simulink model "SpaceRobotics_compare"  (R2024b)
settings: Solver=VariableStepAuto  StartTime=0.0  StopTime=10.0  RelTol=1e-3
values from neighbouring files (symbols this model uses):
  s = joint_angles_new - joint_angles    [inverse_kinematic_broyden.m]
  X = {r0x dr0x r0y dr0y theta0 dtheta0 theta1 dtheta1 theta2 dtheta2}    [Another_derivation_trail.m]
undefined symbols (not defined in the file or in its folder): Y, Z
libraries: sm_lib x23, nesl_utility x9
settings Model: Creator=Daniel  LastModifiedBy=admin

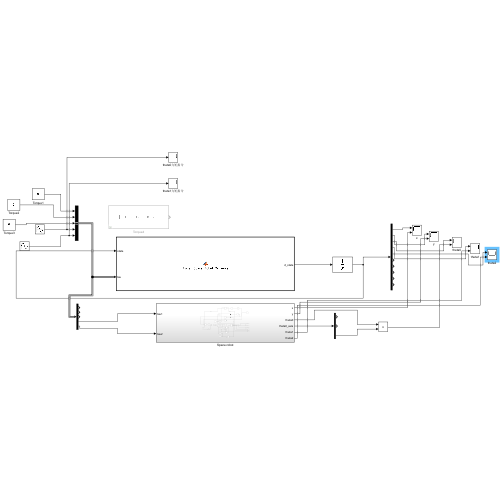
[thumbnail: Simulink's stored preview of the top-level diagram]
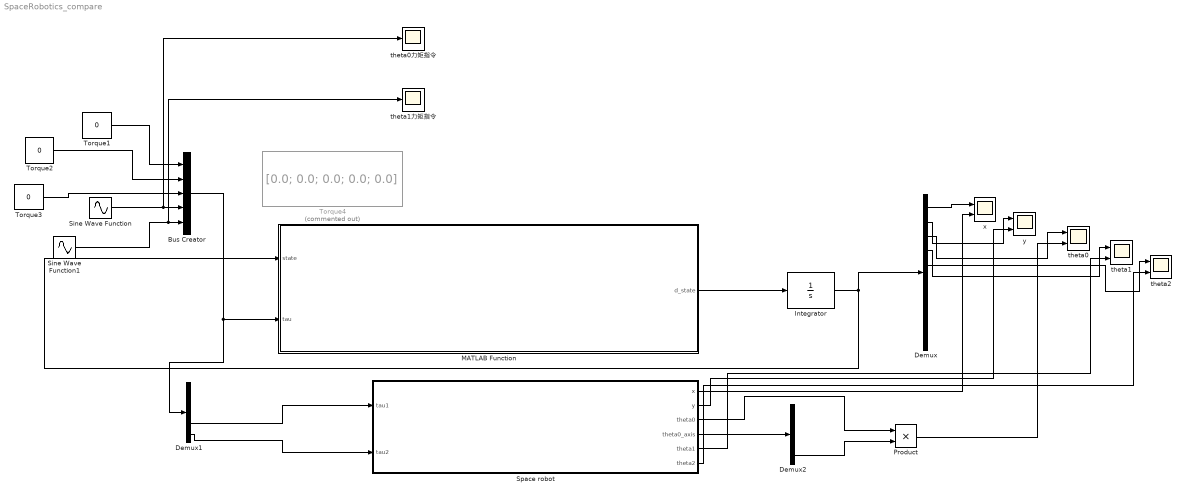
== system SpaceRobotics_compare ==
  Bus Creator : BusCreator  Inputs=5
  Demux : Demux  Outputs=10
  Demux1 : Demux  Outputs=5
  Demux2 : Demux  Outputs=3
  Integrator : Integrator  InitialCondition=[0.0; 0.0; 0.0; 0.0; 0.0; 0.0; 0.0; 0.0; 0.0; 0.0]
  MATLAB Function : MATLAB Function  TreatAsAtomicUnit=on
  Product : Product
  Sine Wave Function : Sin  SampleTime=0
  Sine Wave Function1 : Sin  Phase=pi/2  SampleTime=0
  Space robot : Subsystem
  Torque1 : Constant  Value=0
  Torque2 : Constant  Value=0
  Torque3 : Constant  Value=0
  Torque4 : Constant  Commented=on  Value=[0.0; 0.0; 0.0; 0.0; 0.0]
  theta0 : Scope  NumInputPorts=2
  theta0力矩指令 : Scope
  theta1 : Scope  NumInputPorts=2
  theta1力矩指令 : Scope
  theta2 : Scope  NumInputPorts=2
  x : Scope  NumInputPorts=2
  y : Scope  NumInputPorts=2
  wires:
  MATLAB Function/1(d_state) -> Integrator/1
  Integrator/1 -> MATLAB Function/1(state), Demux/1
  Bus Creator/1 -> Demux1/1, MATLAB Function/2(tau)
  Demux/1 -> x/1
  Demux/2 -> y/1
  Demux/3 -> theta0/1
  Demux/4 -> theta1/1
  Demux/5 -> theta2/1
  Demux1/5 -> Space robot/2(tau2)
  Demux1/4 -> Space robot/1(tau1)
  Space robot/1(x) -> x/2
  Space robot/2(y) -> y/2
  Space robot/5(theta1) -> theta1/2
  Space robot/6(theta2) -> theta2/2
  Torque1/1 -> Bus Creator/1
  Torque2/1 -> Bus Creator/2
  Torque3/1 -> Bus Creator/3
  Sine Wave Function/1 -> theta0力矩指令/1, Bus Creator/4
  Sine Wave Function1/1 -> theta1力矩指令/1, Bus Creator/5
  Space robot/4(theta0_axis) -> Demux2/1
  Demux2/3 -> Product/2
  Space robot/3(theta0) -> Product/1
  Product/1 -> theta0/2

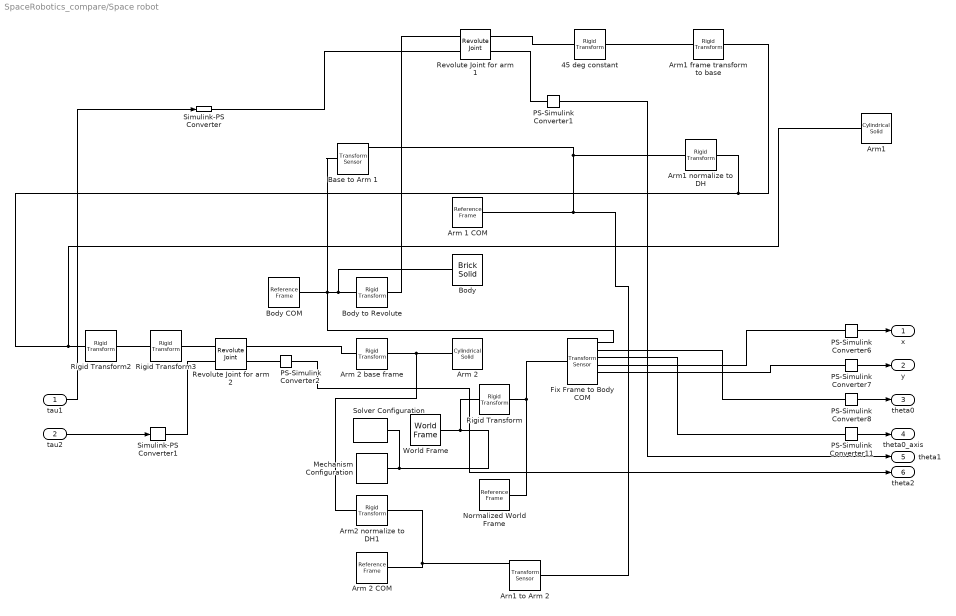
== system SpaceRobotics_compare/Space robot ==
  tau1 : Inport
  tau2 : Inport  Port=2
  45 deg constant : sm_lib/Frames and Transforms/Rigid Transform  RotationMethod=StandardAxis  FollAlignAxisA=+X  BaseAlignAxisA=+Y  FollAlignAxisB=+Y  BaseAlignAxisB=+Z  RotationStandardAxis=+Z  RotationAngle=45  RotationAngleUnits=deg  RotationArbitraryAxis=[0 0 1]  RotationSequenceAxes=FollowerAxes  RotationSequence=XYX  RotationSequenceAngles=[0 0 0]  RotationSequenceAnglesUnits=deg  RotationMatrix=[1 0 0;0 1 0;0 0 1]  Quaternion=[1 0 0 0]  TranslationMethod=Cartesian  TranslationCartesianOffset=[0 0 0]  TranslationCartesianOffsetUnits=m  TranslationStandardAxis=+Z  TranslationStandardOffset=0  TranslationStandardOffsetUnits=m  TranslationROffset=0  TranslationROffsetUnits=m  TranslationThetaOffset=0  TranslationThetaOffsetUnits=deg  TranslationZOffset=0  TranslationZOffsetUnits=m
  Arm 1 COM : sm_lib/Frames and Transforms/Reference Frame
  Arm 2 : sm_lib/Body Elements/Cylindrical Solid  CylinderRadius=0.12  CylinderRadiusUnits=m  CylinderLength=1  CylinderLengthUnits=m  ExportEntireGeometry=off  InertiaType=Custom  BasedOnType=Density  Density=1000  DensityUnits=kg/m^3  Mass=10  MassUnits=kg  CenterOfMass=[0 0 0]  CenterOfMassUnits=m  MomentsOfInertia=[2 2 2]  MomentsOfInertiaUnits=kg*m^2  ProductsOfInertia=[0 0 0]  ProductsOfInertiaUnits=kg*m^2  GraphicType=FromGeometry  MarkerShape=Sphere  MarkerSize=10  GraphicVisPropType=SimpleVisualProperties  GraphicDiffuseColor=[0.5 0.5 0.5]  GraphicOpacity=1  GraphicSpecularColor=[0.5 0.5 0.5 1.0]  GraphicAmbientColor=[0.15 0.15 0.15 1.0]  GraphicEmissiveColor=[0.0 0.0 0.0 1.0]  GraphicShininess=75  DoExposeReferenceFrame=on  SerializedFrames=<Frames/>
  Arm 2 COM : sm_lib/Frames and Transforms/Reference Frame
  Arm 2 base frame : sm_lib/Frames and Transforms/Rigid Transform  RotationMethod=StandardAxis  FollAlignAxisA=+X  BaseAlignAxisA=+Y  FollAlignAxisB=+Y  BaseAlignAxisB=+Z  RotationStandardAxis=+X  RotationAngle=90  RotationAngleUnits=deg  RotationArbitraryAxis=[0 0 1]  RotationSequenceAxes=FollowerAxes  RotationSequence=XYX  RotationSequenceAngles=[0 0 0]  RotationSequenceAnglesUnits=deg  RotationMatrix=[1 0 0;0 1 0;0 0 1]  Quaternion=[1 0 0 0]  TranslationMethod=Cartesian  TranslationCartesianOffset=[0 0 -0.5]  TranslationCartesianOffsetUnits=m  TranslationStandardAxis=+Z  TranslationStandardOffset=0  TranslationStandardOffsetUnits=m  TranslationROffset=0  TranslationROffsetUnits=m  TranslationThetaOffset=0  TranslationThetaOffsetUnits=deg  TranslationZOffset=0  TranslationZOffsetUnits=m
  Arm1 : sm_lib/Body Elements/Cylindrical Solid  CylinderRadius=0.12  CylinderRadiusUnits=m  CylinderLength=1  CylinderLengthUnits=m  ExportEntireGeometry=off  InertiaType=Custom  BasedOnType=Density  Density=1000  DensityUnits=kg/m^3  Mass=10  MassUnits=kg  CenterOfMass=[0 0 0]  CenterOfMassUnits=m  MomentsOfInertia=[2 2 2]  MomentsOfInertiaUnits=kg*m^2  ProductsOfInertia=[0 0 0]  ProductsOfInertiaUnits=kg*m^2  GraphicType=FromGeometry  MarkerShape=Sphere  MarkerSize=10  GraphicVisPropType=SimpleVisualProperties  GraphicDiffuseColor=[0.5 0.5 0.5]  GraphicOpacity=1  GraphicSpecularColor=[0.5 0.5 0.5 1.0]  GraphicAmbientColor=[0.15 0.15 0.15 1.0]  GraphicEmissiveColor=[0.0 0.0 0.0 1.0]  GraphicShininess=75  DoExposeReferenceFrame=on  SerializedFrames=<Frames/>
  Arm1 frame transform to base : sm_lib/Frames and Transforms/Rigid Transform  RotationMethod=StandardAxis  FollAlignAxisA=+X  BaseAlignAxisA=+Y  FollAlignAxisB=+Y  BaseAlignAxisB=+Z  RotationStandardAxis=+X  RotationAngle=90  RotationAngleUnits=deg  RotationArbitraryAxis=[0 0 1]  RotationSequenceAxes=FollowerAxes  RotationSequence=XYX  RotationSequenceAngles=[0 0 0]  RotationSequenceAnglesUnits=deg  RotationMatrix=[1 0 0;0 1 0;0 0 1]  Quaternion=[1 0 0 0]  TranslationMethod=Cartesian  TranslationCartesianOffset=[0 0 -0.5]  TranslationCartesianOffsetUnits=m  TranslationStandardAxis=+Z  TranslationStandardOffset=0  TranslationStandardOffsetUnits=m  TranslationROffset=0  TranslationROffsetUnits=m  TranslationThetaOffset=0  TranslationThetaOffsetUnits=deg  TranslationZOffset=0  TranslationZOffsetUnits=m
  Arm1 normalize to DH : sm_lib/Frames and Transforms/Rigid Transform  RotationMethod=RotationMatrix  FollAlignAxisA=+X  BaseAlignAxisA=+Y  FollAlignAxisB=+Y  BaseAlignAxisB=+Z  RotationStandardAxis=+X  RotationAngle=90  RotationAngleUnits=deg  RotationArbitraryAxis=[0 0 1]  RotationSequenceAxes=FollowerAxes  RotationSequence=XYX  RotationSequenceAngles=[0 0 0]  RotationSequenceAnglesUnits=deg  RotationMatrix=[0 0 1;-1 0 0;0 -1 0]  Quaternion=[1 0 0 0]  TranslationMethod=None  TranslationCartesianOffset=[0 0 0]  TranslationCartesianOffsetUnits=m  TranslationStandardAxis=+Z  TranslationStandardOffset=0  TranslationStandardOffsetUnits=m  TranslationROffset=0  TranslationROffsetUnits=m  TranslationThetaOffset=0  TranslationThetaOffsetUnits=deg  TranslationZOffset=0  TranslationZOffsetUnits=m
  Arm2 normalize to DH1 : sm_lib/Frames and Transforms/Rigid Transform  RotationMethod=RotationMatrix  FollAlignAxisA=+X  BaseAlignAxisA=+Y  FollAlignAxisB=+Y  BaseAlignAxisB=+Z  RotationStandardAxis=+X  RotationAngle=90  RotationAngleUnits=deg  RotationArbitraryAxis=[0 0 1]  RotationSequenceAxes=FollowerAxes  RotationSequence=XYX  RotationSequenceAngles=[0 0 0]  RotationSequenceAnglesUnits=deg  RotationMatrix=[0 0 1;-1 0 0;0 -1 0]  Quaternion=[1 0 0 0]  TranslationMethod=None  TranslationCartesianOffset=[0 0 0]  TranslationCartesianOffsetUnits=m  TranslationStandardAxis=+Z  TranslationStandardOffset=0  TranslationStandardOffsetUnits=m  TranslationROffset=0  TranslationROffsetUnits=m  TranslationThetaOffset=0  TranslationThetaOffsetUnits=deg  TranslationZOffset=0  TranslationZOffsetUnits=m
  Arn1 to Arm 2 : sm_lib/Frames and Transforms/Transform Sensor  MeasurementFrame=Base  RotationSequence=XYX  SenseAngle=on  SenseAxis=on  SenseQ=off  SenseR=off  SenseRotationSequence=off  SenseOmegaX=off  SenseOmegaY=off  SenseOmegaZ=off  SenseOmega=off  SenseQDot=off  SenseRDot=off  SenseRotationSequenceDot=off  SenseAlphaX=off  SenseAlphaY=off  SenseAlphaZ=off  SenseAlpha=off  SenseQDDot=off  SenseRDDot=off  SenseX=off  SenseY=off  SenseZ=off  SenseXYZ=off  SenseRad=off  SenseAzim=off  SenseDist=off  SenseInc=off  SenseXDot=off  SenseYDot=off  SenseZDot=off  SenseXYZDot=off  SenseRadDot=off  SenseAzimDot=off  SenseDistDot=off  SenseIncDot=off  SenseXDDot=off  SenseYDDot=off  SenseZDDot=off  SenseXYZDDot=off  SenseRadDDot=off  SenseAzimDDot=off  SenseDistDDot=off  SenseIncDDot=off
  Base to Arm 1 : sm_lib/Frames and Transforms/Transform Sensor  MeasurementFrame=Base  RotationSequence=XYX  SenseAngle=on  SenseAxis=on  SenseQ=off  SenseR=off  SenseRotationSequence=off  SenseOmegaX=off  SenseOmegaY=off  SenseOmegaZ=off  SenseOmega=off  SenseQDot=off  SenseRDot=off  SenseRotationSequenceDot=off  SenseAlphaX=off  SenseAlphaY=off  SenseAlphaZ=off  SenseAlpha=off  SenseQDDot=off  SenseRDDot=off  SenseX=off  SenseY=off  SenseZ=off  SenseXYZ=off  SenseRad=off  SenseAzim=off  SenseDist=off  SenseInc=off  SenseXDot=off  SenseYDot=off  SenseZDot=off  SenseXYZDot=off  SenseRadDot=off  SenseAzimDot=off  SenseDistDot=off  SenseIncDot=off  SenseXDDot=off  SenseYDDot=off  SenseZDDot=off  SenseXYZDDot=off  SenseRadDDot=off  SenseAzimDDot=off  SenseDistDDot=off  SenseIncDDot=off
  Body : sm_lib/Body Elements/Brick Solid  BrickDimensions=[1 1 1]  BrickDimensionsUnits=m  ExportEntireGeometry=off  InertiaType=CalculateFromGeometry  BasedOnType=Density  Density=500  DensityUnits=kg/m^3  Mass=1  MassUnits=kg  CenterOfMass=[0 0 0]  CenterOfMassUnits=m  MomentsOfInertia=[1 1 1]  MomentsOfInertiaUnits=kg*m^2  ProductsOfInertia=[0 0 0]  ProductsOfInertiaUnits=kg*m^2  GraphicType=FromGeometry  MarkerShape=Sphere  MarkerSize=10  GraphicVisPropType=SimpleVisualProperties  GraphicDiffuseColor=[0.5 0.5 0.5]  GraphicOpacity=1  GraphicSpecularColor=[0.5 0.5 0.5 1.0]  GraphicAmbientColor=[0.15 0.15 0.15 1.0]  GraphicEmissiveColor=[0.0 0.0 0.0 1.0]  GraphicShininess=75  DoExposeReferenceFrame=on  SerializedFrames=<Frames><Frame><Id>Frame1</Id><Value><Name>F1</Name><Origin><Source>CenterOfMassFrame</Source><FeatureName></FeatureName></Origin><PrimaryAxis><DefinedDirection>+Z</DefinedDirection><Source>ReferenceFrame</Source><SourceDirection>+Z</SourceDirection><FeatureName></FeatureName></PrimaryAxis><SecondaryAxis><DefinedDirection>+X</DefinedDirection><Source>ReferenceFrame</Source><SourceDirection>+X</SourceDirection><FeatureName></FeatureName></SecondaryAxis></Value></Frame></Frames>
  Body COM : sm_lib/Frames and Transforms/Reference Frame
  Body to Revolute : sm_lib/Frames and Transforms/Rigid Transform  RotationMethod=None  FollAlignAxisA=+X  BaseAlignAxisA=+Y  FollAlignAxisB=+Y  BaseAlignAxisB=+Z  RotationStandardAxis=+X  RotationAngle=90  RotationAngleUnits=deg  RotationArbitraryAxis=[0 0 1]  RotationSequenceAxes=FollowerAxes  RotationSequence=XYX  RotationSequenceAngles=[0 0 0]  RotationSequenceAnglesUnits=deg  RotationMatrix=[1 0 0;0 1 0;0 0 1]  Quaternion=[1 0 0 0]  TranslationMethod=Cartesian  TranslationCartesianOffset=[0.5 0.5 0]  TranslationCartesianOffsetUnits=m  TranslationStandardAxis=+Z  TranslationStandardOffset=0  TranslationStandardOffsetUnits=m  TranslationROffset=0  TranslationROffsetUnits=m  TranslationThetaOffset=0  TranslationThetaOffsetUnits=deg  TranslationZOffset=0  TranslationZOffsetUnits=m
  Fix Frame to Body COM : sm_lib/Frames and Transforms/Transform Sensor  MeasurementFrame=World  RotationSequence=XYX  SenseAngle=on  SenseAxis=on  SenseQ=off  SenseR=off  SenseRotationSequence=off  SenseOmegaX=off  SenseOmegaY=off  SenseOmegaZ=off  SenseOmega=off  SenseQDot=off  SenseRDot=off  SenseRotationSequenceDot=off  SenseAlphaX=off  SenseAlphaY=off  SenseAlphaZ=off  SenseAlpha=off  SenseQDDot=off  SenseRDDot=off  SenseX=on  SenseY=on  SenseZ=off  SenseXYZ=on  SenseRad=off  SenseAzim=off  SenseDist=off  SenseInc=off  SenseXDot=off  SenseYDot=off  SenseZDot=off  SenseXYZDot=off  SenseRadDot=off  SenseAzimDot=off  SenseDistDot=off  SenseIncDot=off  SenseXDDot=off  SenseYDDot=off  SenseZDDot=off  SenseXYZDDot=off  SenseRadDDot=off  SenseAzimDDot=off  SenseDistDDot=off  SenseIncDDot=off
  Mechanism Configuration : sm_lib/Utilities/Mechanism Configuration  UniformGravity=Constant  GravityVector=[0 0 0]  GravityVectorUnits=m/s^2  LinearizationDelta=0.001  JointModeTransitionNonlinearIterations=100
  Normalized World Frame : sm_lib/Frames and Transforms/Reference Frame
  PS-Simulink Converter{1..2,6..8,11} (6 alike) : nesl_utility/PS-Simulink Converter  PhysicalDomain=network_engine_domain  SubClassName=ps_output  LeftPortType=input  RightPortType=output  PseudoPeriodic=off  Frequencies=[]  VectorFormat=inherit  Unit=inherit  AffineConversion=off
  Revolute Joint for arm 1 : sm_lib/Joints/Revolute Joint  JointMode=Normal  CompositeWrenchDir=BaseOnFollower  CompositeWrenchFrame=BaseFrame  SenseConstraintForce=off  SenseConstraintTorque=off  SenseTotalForce=off  SenseTotalTorque=off  PositionTargetSpecify=on  PositionTargetPriority=High  PositionTargetValue=0  PositionTargetValueUnits=deg  VelocityTargetSpecify=off  VelocityTargetPriority=High  VelocityTargetValue=0  VelocityTargetValueUnits=deg/s  EquilibriumPosition=0  EquilibriumPositionUnits=deg  SpringStiffness=0  SpringStiffnessUnits=N*m/deg  DampingCoefficient=0  DampingCoefficientUnits=N*m/(deg/s)  LowerLimitSpecify=off  LowerLimitBound=-90  LowerLimitBoundUnits=deg  LowerLimitStiffness=1e4  LowerLimitStiffnessUnits=N*m/deg  LowerLimitDamping=10  LowerLimitDampingUnits=N*m/(deg/s)  LowerLimitTransitionRegionWidth=0.1  LowerLimitTransitionRegionWidthUnits=deg  UpperLimitSpecify=off  UpperLimitBound=90  UpperLimitBoundUnits=deg  UpperLimitStiffness=1e4  UpperLimitStiffnessUnits=N*m/deg  UpperLimitDamping=10  UpperLimitDampingUnits=N*m/(deg/s)  UpperLimitTransitionRegionWidth=0.1  UpperLimitTransitionRegionWidthUnits=deg  TorqueActuationMode=InputTorque  MotionActuationMode=ComputedMotion  SensePosition=on  SenseVelocity=off  SenseAcceleration=off  SenseTorqueForce=off  SenseLowerLimitTorqueForce=off  SenseUpperLimitTorqueForce=off
  Revolute Joint for arm 2 : sm_lib/Joints/Revolute Joint  JointMode=Normal  CompositeWrenchDir=BaseOnFollower  CompositeWrenchFrame=BaseFrame  SenseConstraintForce=off  SenseConstraintTorque=off  SenseTotalForce=off  SenseTotalTorque=off  PositionTargetSpecify=on  PositionTargetPriority=High  PositionTargetValue=0  PositionTargetValueUnits=deg  VelocityTargetSpecify=off  VelocityTargetPriority=High  VelocityTargetValue=0  VelocityTargetValueUnits=deg/s  EquilibriumPosition=0  EquilibriumPositionUnits=deg  SpringStiffness=0  SpringStiffnessUnits=N*m/deg  DampingCoefficient=0  DampingCoefficientUnits=N*m/(deg/s)  LowerLimitSpecify=off  LowerLimitBound=-90  LowerLimitBoundUnits=deg  LowerLimitStiffness=1e4  LowerLimitStiffnessUnits=N*m/deg  LowerLimitDamping=10  LowerLimitDampingUnits=N*m/(deg/s)  LowerLimitTransitionRegionWidth=0.1  LowerLimitTransitionRegionWidthUnits=deg  UpperLimitSpecify=off  UpperLimitBound=90  UpperLimitBoundUnits=deg  UpperLimitStiffness=1e4  UpperLimitStiffnessUnits=N*m/deg  UpperLimitDamping=10  UpperLimitDampingUnits=N*m/(deg/s)  UpperLimitTransitionRegionWidth=0.1  UpperLimitTransitionRegionWidthUnits=deg  TorqueActuationMode=InputTorque  MotionActuationMode=ComputedMotion  SensePosition=on  SenseVelocity=off  SenseAcceleration=off  SenseTorqueForce=off  SenseLowerLimitTorqueForce=off  SenseUpperLimitTorqueForce=off
  Rigid Transform : sm_lib/Frames and Transforms/Rigid Transform  RotationMethod=StandardAxis  FollAlignAxisA=+X  BaseAlignAxisA=+Y  FollAlignAxisB=+Y  BaseAlignAxisB=+Z  RotationStandardAxis=+Z  RotationAngle=-45  RotationAngleUnits=deg  RotationArbitraryAxis=[0 0 1]  RotationSequenceAxes=FollowerAxes  RotationSequence=XYX  RotationSequenceAngles=[0 0 0]  RotationSequenceAnglesUnits=deg  RotationMatrix=[1 0 0;0 1 0;0 0 1]  Quaternion=[1 0 0 0]  TranslationMethod=Cartesian  TranslationCartesianOffset=[-1.20711 0 0]  TranslationCartesianOffsetUnits=m  TranslationStandardAxis=+Z  TranslationStandardOffset=0  TranslationStandardOffsetUnits=m  TranslationROffset=0  TranslationROffsetUnits=m  TranslationThetaOffset=0  TranslationThetaOffsetUnits=deg  TranslationZOffset=0  TranslationZOffsetUnits=m
  Rigid Transform2 : sm_lib/Frames and Transforms/Rigid Transform  RotationMethod=StandardAxis  FollAlignAxisA=+X  BaseAlignAxisA=+Y  FollAlignAxisB=+Y  BaseAlignAxisB=+Z  RotationStandardAxis=+Z  RotationAngle=0  RotationAngleUnits=deg  RotationArbitraryAxis=[0 0 1]  RotationSequenceAxes=FollowerAxes  RotationSequence=XYX  RotationSequenceAngles=[0 0 0]  RotationSequenceAnglesUnits=deg  RotationMatrix=[1 0 0;0 1 0;0 0 1]  Quaternion=[1 0 0 0]  TranslationMethod=Cartesian  TranslationCartesianOffset=[0 0 0.5]  TranslationCartesianOffsetUnits=m  TranslationStandardAxis=+Z  TranslationStandardOffset=0  TranslationStandardOffsetUnits=m  TranslationROffset=0  TranslationROffsetUnits=m  TranslationThetaOffset=0  TranslationThetaOffsetUnits=deg  TranslationZOffset=0  TranslationZOffsetUnits=m
  Rigid Transform3 : sm_lib/Frames and Transforms/Rigid Transform  RotationMethod=StandardAxis  FollAlignAxisA=+X  BaseAlignAxisA=+Y  FollAlignAxisB=+Y  BaseAlignAxisB=+Z  RotationStandardAxis=+X  RotationAngle=90  RotationAngleUnits=deg  RotationArbitraryAxis=[0 0 1]  RotationSequenceAxes=FollowerAxes  RotationSequence=XYX  RotationSequenceAngles=[0 0 0]  RotationSequenceAnglesUnits=deg  RotationMatrix=[1 0 0;0 1 0;0 0 1]  Quaternion=[1 0 0 0]  TranslationMethod=Cartesian  TranslationCartesianOffset=[0 0 0]  TranslationCartesianOffsetUnits=m  TranslationStandardAxis=+Z  TranslationStandardOffset=0  TranslationStandardOffsetUnits=m  TranslationROffset=0  TranslationROffsetUnits=m  TranslationThetaOffset=0  TranslationThetaOffsetUnits=deg  TranslationZOffset=0  TranslationZOffsetUnits=m
  Simulink-PS Converter : nesl_utility/Simulink-PS Converter  PhysicalDomain=network_engine_domain  SubClassName=ps_input  LeftPortType=input  RightPortType=output  PseudoPeriodic=off  Frequencies=[]  NoiseDistribution=none  NoiseParameters=[]  Unit=1  AffineConversion=off  FilteringAndDerivatives=provide  SimscapeFilterOrder=1  InputFilterTimeConstant=0.001  UdotUserProvided=0
  Simulink-PS Converter1 : nesl_utility/Simulink-PS Converter  PhysicalDomain=network_engine_domain  SubClassName=ps_input  LeftPortType=input  RightPortType=output  PseudoPeriodic=off  Frequencies=[]  NoiseDistribution=none  NoiseParameters=[]  Unit=1  AffineConversion=off  FilteringAndDerivatives=provide  SimscapeFilterOrder=1  InputFilterTimeConstant=0.001  UdotUserProvided=0
  Solver Configuration : nesl_utility/Solver Configuration  PhysicalDomain=network_engine_domain  SubClassName=solver  LeftPortType=input  RightPortType=generic  Tones=[]  Harmonics=[]  SimulateNoise=off  Profile=off  UseLocalSampling=off  EnableSwitchedLinearOptims=on  FrequencyDomain=off  UseCCode=off  RelTol=0.001  AbsTol=0.001  MinStep=1e-09  ToWorkspace=off  RevertToSquareIcSolve=off  NumHomotopyIterations=100  PhasorMode=off  PhasorModeNumHarmonics=1  ConsistencySolver=NEWTON_XTOL_AFTER_FTOL  IndexReductionMethod=DerivativeReplacement  DoDC=off  ResidualTolerance=1e-09  ConsistencyTolSource=GLOBAL  ConsistencyAbsTol=0.001  ConsistencyRelTol=0.001  ConsistencyTolFactor=0.001  UseLocalSolver=off  LocalSolverChoice=NE_BACKWARD_EULER_ADVANCER  ResolveIndetEquations=on  FunctionEvalNumThread=1  LocalSolverSampleTime=0.001  DoFixedCost=off  MaxNonlinIter=3  MaxModeIter=2  ComputeImpulses=off  ImpulseIterations=2  LinearAlgebra=auto  LinearAlgebraNumThread=0  EquationFormulation=NE_TIME_EF  DelaysMemoryBudget=1024  AutomaticFiltering=on  FilteringTimeConstant=0.001  PartitionStorageMethod=AS_NEEDED  PartitionMemoryBudget=1024  PartitionMethod=ROBUST  MultibodyUseLocalSolver=off  MultibodyLocalSolverChoice=ODE1  MultibodyLocalSolverSampleTime=0.001
  World Frame : sm_lib/Frames and Transforms/World Frame
  x : Outport
  y : Outport  Port=2
  theta0 : Outport  Port=3
  theta0_axis : Outport  Port=4
  theta1 : Outport  Port=5
  theta2 : Outport  Port=6
  wires:
  PS-Simulink Converter1/1 -> theta1/1
  tau2/1 -> Simulink-PS Converter1/1
  tau1/1 -> Simulink-PS Converter/1
  PS-Simulink Converter7/1 -> y/1
  PS-Simulink Converter8/1 -> theta0/1
  PS-Simulink Converter11/1 -> theta0_axis/1
  PS-Simulink Converter6/1 -> x/1
  PS-Simulink Converter2/1 -> theta2/1
  connections:
  Rigid Transform3/RConn1 -- Revolute Joint for arm 2/LConn1
  Arn1 to Arm 2/LConn1 -- Arm 1 COM/RConn1 -- Arm1 normalize to DH/LConn1 -- Base to Arm 1/RConn1
  Revolute Joint for arm 2/RConn1 -- Arm 2 base frame/RConn1
  Arm1/RConn1 -- Arm1 frame transform to base/LConn1 -- Arm1 normalize to DH/RConn1 -- Rigid Transform2/LConn1
  Rigid Transform2/RConn1 -- Rigid Transform3/LConn1
  PS-Simulink Converter6/LConn1 -- Fix Frame to Body COM/RConn4
  PS-Simulink Converter7/LConn1 -- Fix Frame to Body COM/RConn5
  Simulink-PS Converter/RConn1 -- Revolute Joint for arm 1/LConn2
  Simulink-PS Converter1/RConn1 -- Revolute Joint for arm 2/LConn2
  Body to Revolute/LConn1 -- Base to Arm 1/LConn1 -- Body COM/RConn1 -- Fix Frame to Body COM/RConn1 -- Body/RConn1
  Arm2 normalize to DH1/LConn1 -- Arm 2 COM/RConn1 -- Arn1 to Arm 2/RConn1
  Revolute Joint for arm 1/RConn2 -- PS-Simulink Converter1/LConn1
  World Frame/RConn1 -- Solver Configuration/RConn1 -- Mechanism Configuration/RConn1 -- Rigid Transform/LConn1
  Rigid Transform/RConn1 -- Fix Frame to Body COM/LConn1 -- Normalized World Frame/RConn1
  PS-Simulink Converter8/LConn1 -- Fix Frame to Body COM/RConn2
  Body to Revolute/RConn1 -- Revolute Joint for arm 1/LConn1
  Arm 2 base frame/LConn1 -- Arm2 normalize to DH1/RConn1 -- Arm 2/RConn1
  Revolute Joint for arm 1/RConn1 -- 45 deg constant/RConn1
  45 deg constant/LConn1 -- Arm1 frame transform to base/RConn1
  Fix Frame to Body COM/RConn3 -- PS-Simulink Converter11/LConn1
  PS-Simulink Converter2/LConn1 -- Revolute Joint for arm 2/RConn2

== matlab function SpaceRobotics_compare/MATLAB Function ==
  data: d_state output; state input; tau input
function d_state = Planar_Space_Robot_Dynamics(state, tau)
    % Explicit definition of dynamic constants
    robot_dynamics_constants.m0 = 500;
    robot_dynamics_constants.m1 = 10;
    robot_dynamics_constants.m2 = 10;
    robot_dynamics_constants.b0 = sqrt(0.5^2 + 0.5^2);
    robot_dynamics_constants.l1 = 1;
    robot_dynamics_constants.l2 = 1;
    robot_dynamics_constants.Ic0 = 83.3333;
    robot_dynamics_constants.Ic1 = 2;
    robot_dynamics_constants.Ic2 = 2;

    normalized_theta0 = mod(state(3), 2*pi);
    normalized_theta1 = mod(state(4), 2*pi);
    normalized_theta2 = mod(state(5), 2*pi);
    q = state(1:5);
    q(3) = normalized_theta0;
    q(4) = normalized_theta1;
    q(5) = normalized_theta2;
    q_dot = state(6:10);
    
    [inertial_term_matrix, coriolis_term] = Get_Planar_Dynamic_Matrix(q, q_dot, robot_dynamics_constants);
    %Dq = tau - coriolis_term;
    Dq = tau - coriolis_term;

    q_ddot = inertial_term_matrix \ Dq;

    d_state = [q_dot; q_ddot];
end

% Man fuck finally it matches hahahahahahahaha

function [H, F] = Get_Planar_Dynamic_Matrix(state_vector, state_dot, robot_dynamics_constants)
    % state_vector = [r0x, r0y, theta0, theta1, theta2]
    % state_dot = [r0x_dot, r0y_dot, theta0_dot, theta1_dot, theta2_dot]
    % Planar space robot dynamics
    % angles
    theta0 = state_vector(3);
    theta1 = state_vector(4);
    theta2 = state_vector(5);
    theta0_dot = state_dot(3);
    theta1_dot = state_dot(4);
    theta2_dot = state_dot(5);
    c0 = cos(theta0);
    c1 = cos(theta1);
    c2 = cos(theta2);
    c01 = cos(theta0 + theta1);
    c02 = cos(theta0 + theta2);
    c12 = cos(theta1 + theta2);
    c012 = cos(theta0 + theta1 + theta2);
    s0 = sin(theta0);
    s1 = sin(theta1);
    s2 = sin(theta2);
    s01 = sin(theta0 + theta1);
    s02 = sin(theta0 + theta2);
    s12 = sin(theta1 + theta2);
    s012 = sin(theta0 + theta1 + theta2);

    m_0 = robot_dynamics_constants.m0;
    m_1 = robot_dynamics_constants.m1;
    m_2 = robot_dynamics_constants.m2;
    b_0 = robot_dynamics_constants.b0;
    l_1 = robot_dynamics_constants.l1;
    l_2 = robot_dynamics_constants.l2;
    I_c0 = robot_dynamics_constants.Ic0;
    I_c1 = robot_dynamics_constants.Ic1;
    I_c2 = robot_dynamics_constants.Ic2;



    % Define the h matrix elements based on the equations provided
    h11 = m_0 + m_1 + m_2;
    h12 = 0;
    h13 = - (m_1*(2*b_0*s0 + l_1*s01))/2 - (m_2*(2*b_0*s0 + 2*l_1*s01 + l_2*s012))/2;
    h14 = - (m_2*(2*l_1*s01 + l_2*s012))/2 - (l_1*m_1*s01)/2;
    h15 = -(l_2*m_2*s012)/2;
    
    h21 = 0;
    h22 = m_0 + m_1 + m_2;
    h23 = (m_1*(2*b_0*c0 + c01*l_1))/2 + (m_2*(2*b_0*c0 + 2*c01*l_1 + c012*l_2))/2;
    h24 = (m_2*(2*c01*l_1 + c012*l_2))/2 + (c01*l_1*m_1)/2;
    h25 = (c012*l_2*m_2)/2;
    
    h31 = - m_1*(b_0*s0 + (l_1*s01)/2) - m_2*(b_0*s0 + l_1*s01 + (l_2*s012)/2);
    h32 = m_1*(b_0*c0 + (c01*l_1)/2) + m_2*(b_0*c0 + c01*l_1 + (c012*l_2)/2);
    h33 = I_c0 + I_c1 + I_c2 + m_2*(b_0*c0 + c01*l_1 + (c012*l_2)/2)^2 + m_2*(b_0*s0 + l_1*s01 + (l_2*s012)/2)^2 + m_1*(b_0*c0 + (c01*l_1)/2)^2 + m_1*(b_0*s0 + (l_1*s01)/2)^2;
    h34 = I_c1 + I_c2 + m_2*(c01*l_1 + (c012*l_2)/2)*(b_0*c0 + c01*l_1 + (c012*l_2)/2) + m_2*(l_1*s01 + (l_2*s012)/2)*(b_0*s0 + l_1*s01 + (l_2*s012)/2) + (c01*l_1*m_1*(b_0*c0 + (c01*l_1)/2))/2 + (l_1*m_1*s01*(b_0*s0 + (l_1*s01)/2))/2;
    h35 = I_c2 + (c012*l_2*m_2*(b_0*c0 + c01*l_1 + (c012*l_2)/2))/2 + (l_2*m_2*s012*(b_0*s0 + l_1*s01 + (l_2*s012)/2))/2;
    
    h41 = - m_2*(l_1*s01 + (l_2*s012)/2) - (l_1*m_1*s01)/2;
    h42 = m_2*(c01*l_1 + (c012*l_2)/2) + (c01*l_1*m_1)/2;
    h43 = I_c1 + I_c2 + m_2*(c01*l_1 + (c012*l_2)/2)*(b_0*c0 + c01*l_1 + (c012*l_2)/2) + m_2*(l_1*s01 + (l_2*s012)/2)*(b_0*s0 + l_1*s01 + (l_2*s012)/2) + (c01*l_1*m_1*(b_0*c0 + (c01*l_1)/2))/2 + (l_1*m_1*s01*(b_0*s0 + (l_1*s01)/2))/2;
    h44 = I_c1 + I_c2 + m_2*(l_1*s01 + (l_2*s012)/2)^2 + m_2*(c01*l_1 + (c012*l_2)/2)^2 + (c01^2*l_1^2*m_1)/4 + (l_1^2*m_1*s01^2)/4;
    h45 = I_c2 + (c012*l_2*m_2*(c01*l_1 + (c012*l_2)/2))/2 + (l_2*m_2*s012*(l_1*s01 + (l_2*s012)/2))/2;
    
    h51 = -(l_2*m_2*s012)/2;
    h52 = (c012*l_2*m_2)/2;
    h53 = I_c2 + (c012*l_2*m_2*(b_0*c0 + c01*l_1 + (c012*l_2)/2))/2 + (l_2*m_2*s012*(b_0*s0 + l_1*s01 + (l_2*s012)/2))/2;
    h54 = I_c2 + (c012*l_2*m_2*(c01*l_1 + (c012*l_2)/2))/2 + (l_2*m_2*s012*(l_1*s01 + (l_2*s012)/2))/2;
    h55 = (m_2*c012^2*l_2^2)/4 + (m_2*l_2^2*s012^2)/4 + I_c2;
    
    F = [                                                                                                                                                                                                                                                                                                                                                                                                                                                                                                                                                                     - b_0*c0*m_1*theta0_dot^2 - b_0*c0*m_2*theta0_dot^2 - (c01*l_1*m_1*theta0_dot^2)/2 - (c01*l_1*m_1*theta1_dot^2)/2 - c01*l_1*m_2*theta0_dot^2 - c01*l_1*m_2*theta1_dot^2 - (c012*l_2*m_2*theta0_dot^2)/2 - (c012*l_2*m_2*theta1_dot^2)/2 - (c012*l_2*m_2*theta2_dot^2)/2 - c01*l_1*m_1*theta0_dot*theta1_dot - 2*c01*l_1*m_2*theta0_dot*theta1_dot - c012*l_2*m_2*theta0_dot*theta1_dot - c012*l_2*m_2*theta0_dot*theta2_dot - c012*l_2*m_2*theta1_dot*theta2_dot
                                                                                                                                                                                                                                                                                                                                                                                                                                                                                                                                                                     - b_0*m_1*s0*theta0_dot^2 - b_0*m_2*s0*theta0_dot^2 - (l_1*m_1*s01*theta0_dot^2)/2 - (l_1*m_1*s01*theta1_dot^2)/2 - l_1*m_2*s01*theta0_dot^2 - l_1*m_2*s01*theta1_dot^2 - (l_2*m_2*s012*theta0_dot^2)/2 - (l_2*m_2*s012*theta1_dot^2)/2 - (l_2*m_2*s012*theta2_dot^2)/2 - l_1*m_1*s01*theta0_dot*theta1_dot - 2*l_1*m_2*s01*theta0_dot*theta1_dot - l_2*m_2*s012*theta0_dot*theta1_dot - l_2*m_2*s012*theta0_dot*theta2_dot - l_2*m_2*s012*theta1_dot*theta2_dot
(b_0*c01*l_1*m_1*s0*theta1_dot^2)/2 - (b_0*c0*l_1*m_1*s01*theta1_dot^2)/2 - b_0*c0*l_1*m_2*s01*theta1_dot^2 + b_0*c01*l_1*m_2*s0*theta1_dot^2 - (b_0*c0*l_2*m_2*s012*theta1_dot^2)/2 + (b_0*c012*l_2*m_2*s0*theta1_dot^2)/2 - (b_0*c0*l_2*m_2*s012*theta2_dot^2)/2 + (b_0*c012*l_2*m_2*s0*theta2_dot^2)/2 - (c01*l_1*l_2*m_2*s012*theta2_dot^2)/2 + (c012*l_1*l_2*m_2*s01*theta2_dot^2)/2 - b_0*c0*l_1*m_1*s01*theta0_dot*theta1_dot + b_0*c01*l_1*m_1*s0*theta0_dot*theta1_dot - 2*b_0*c0*l_1*m_2*s01*theta0_dot*theta1_dot + 2*b_0*c01*l_1*m_2*s0*theta0_dot*theta1_dot - b_0*c0*l_2*m_2*s012*theta0_dot*theta1_dot + b_0*c012*l_2*m_2*s0*theta0_dot*theta1_dot - b_0*c0*l_2*m_2*s012*theta0_dot*theta2_dot + b_0*c012*l_2*m_2*s0*theta0_dot*theta2_dot - b_0*c0*l_2*m_2*s012*theta1_dot*theta2_dot + b_0*c012*l_2*m_2*s0*theta1_dot*theta2_dot - c01*l_1*l_2*m_2*s012*theta0_dot*theta2_dot + c012*l_1*l_2*m_2*s01*theta0_dot*theta2_dot - c01*l_1*l_2*m_2*s012*theta1_dot*theta2_dot + c012*l_1*l_2*m_2*s01*theta1_dot*theta2_dot
                                                                                                                                                                                                                                                                                                                                                                                                                                                                                                                                                                                                                                                                                                                                                                                                                     (b_0*l_1*m_1*s1*theta0_dot^2)/2 + b_0*l_1*m_2*s1*theta0_dot^2 + (b_0*l_2*m_2*s12*theta0_dot^2)/2 - (l_1*l_2*m_2*s2*theta2_dot^2)/2 - l_1*l_2*m_2*s2*theta0_dot*theta2_dot - l_1*l_2*m_2*s2*theta1_dot*theta2_dot
                                                                                                                                                                                                                                                                                                                                                                                                                                                                                                                                                                                                                                                                                                                                                                                                                                                                                                                      (l_2*m_2*(b_0*s12*theta0_dot^2 + l_1*s2*theta0_dot^2 + l_1*s2*theta1_dot^2 + 2*l_1*s2*theta0_dot*theta1_dot))/2];

    
    % Display h and f matrices
    H = [h11, h12, h13, h14, h15;
         h21, h22, h23, h24, h25;
         h31, h32, h33, h34, h35;
         h41, h42, h43, h44, h45;
         h51, h52, h53, h54, h55];
    % F = [f1; f2; f3; f4; f5];
end
